simulink model "AAI_VVI"  (R2020a)
settings: Solver=FixedStepAuto  StartTime=0.0  StopTime=10.0  FixedStep=1e-3  RelTol=1e-3  EnableMultiTasking=on
settings Model: NumberOfSteps=10  PacingRate=0.100000  ExtModeTrigDuration=5  Creator=theodor  LastModifiedBy=theodor
settings OptimizationCC: EnhancedBackFolding=on  PassReuseOutputArgsAs=Individual arguments  ZeroExternalMemoryAtStartup=off  ZeroInternalMemoryAtStartup=off  MaxStackSize=64  OptimizeBlockOrder=speed  DifferentSizesBufferReuse=on  OptimizationCustomize=off  EfficientTunableParamExpr=on
settings DebuggingCC: ParameterTunabilityLossMsg=error
settings HardwareCC: ProdBitPerPointer=32  ProdBitPerSizeT=32  ProdBitPerPtrDiffT=32  ProdLargestAtomicInteger=Long  ProdLargestAtomicFloat=Double  ProdWordSize=32  ProdHWDeviceType=ARM Compatible->ARM Cortex
settings SFSimCC: MATLABDynamicMemAlloc=off
settings RTWCC: SystemTargetFile=ert.tlc  HardwareBoard=NXP FRDM-K64F  TemplateMakefile=ert_default_tmf  Toolchain=GNU Tools for ARM Embedded Processors
settings CodeAppCC: ForceParamTrailComments=on  IgnoreCustomStorageClasses=off  OperatorAnnotations=on  SimulinkDataObjDesc=on  SFDataObjDesc=on  InsertBlockDesc=on

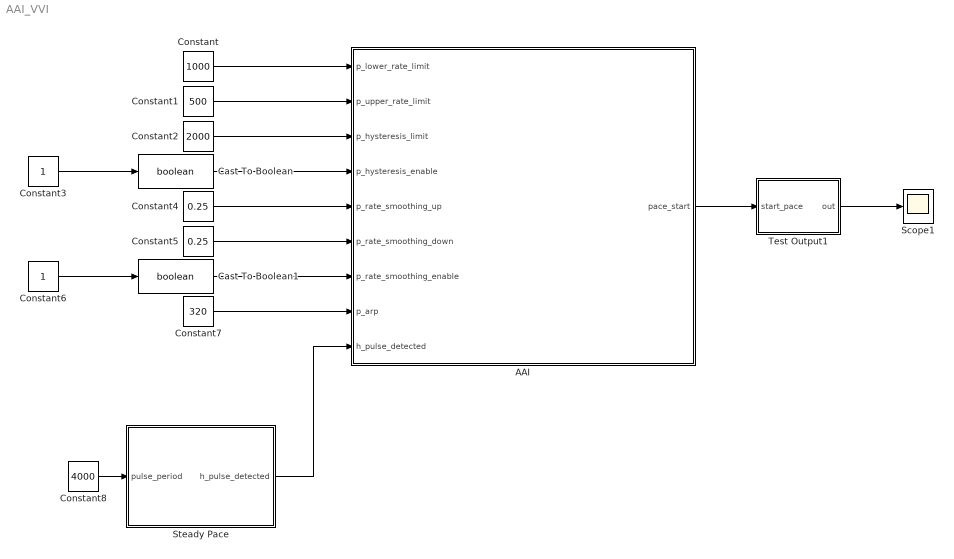
== system AAI_VVI ==
  AAI : Stateflow chart  TreatAsAtomicUnit=on
  Cast To Boolean : DataTypeConversion  OutDataTypeStr=boolean
  Cast To Boolean1 : DataTypeConversion  OutDataTypeStr=boolean
  Constant : Constant  Value=1000
  Constant1 : Constant  Value=500
  Constant2 : Constant  Value=2000
  Constant3 : Constant
  Constant4 : Constant  Value=0.25
  Constant5 : Constant  Value=0.25
  Constant6 : Constant
  Constant7 : Constant  Value=320
  Constant8 : Constant  Value=4000
  Scope1 : Scope
  Steady Pace : Stateflow chart  TreatAsAtomicUnit=on
  Test Output1 : Stateflow chart  TreatAsAtomicUnit=on
  wires:
  Constant/1 -> AAI/1(p_lower_rate_limit)
  Constant1/1 -> AAI/2(p_upper_rate_limit)
  Constant2/1 -> AAI/3(p_hysteresis_limit)
  Constant4/1 -> AAI/5(p_rate_smoothing_up)
  Constant5/1 -> AAI/6(p_rate_smoothing_down)
  Constant7/1 -> AAI/8(p_arp)
  Constant8/1 -> Steady Pace/1(pulse_period)
  Constant3/1 -> Cast To Boolean/1
  Cast To Boolean/1 -> AAI/4(p_hysteresis_enable)
  Constant6/1 -> Cast To Boolean1/1
  Cast To Boolean1/1 -> AAI/7(p_rate_smoothing_enable)
  Test Output1/1(out) -> Scope1/1
  AAI/1(pace_start) -> Test Output1/1(start_pace)
  Steady Pace/1(h_pulse_detected) -> AAI/9(h_pulse_detected)

== stateflow chart AAI_VVI/Steady Pace ==
  state IDLE
    entry:
    h_pulse_detected=false;
  state ON
    entry:
    h_pulse_detected=true;
  (default) -> IDLE
  IDLE -> ON : after(pulse_period-10,msec)
  ON -> IDLE : after(10,msec)
  data: pulse_period input; h_pulse_detected output boolean

== stateflow chart AAI_VVI/AAI ==
  state UPPER_RATE_LIMIT
    entry:
    i_limit = p_upper_rate_limit;
    i_limit = i_limit - p_arp;
    exit: i_last_period = p_arp + elapsed(msec);
  state SENSED
  state LOWER_RATE_LIMIT
    entry:
    i_limit = p_lower_rate_limit;
    i_limit = i_limit - p_arp;
    exit: i_last_period = p_arp + elapsed(msec);
  state INITIAL
    entry:
    i_limit = i_last_period;
  state HYSTERESIS_LIMIT
    entry:
    i_limit = p_hysteresis_limit;
    i_limit = i_limit - p_arp;
    exit: i_last_period = p_arp + elapsed(msec);
  state RATE_SMOOTHING_DOWN
    entry:
    i_limit = i_last_period/(1-p_rate_smoothing_down);
    i_limit = i_limit - p_arp;
    exit: i_last_period = p_arp + elapsed(msec);
  state PACED
    entry:
    pace_start = 1;
    on after(1,msec):
    pace_start = 0;
  state RATE_SMOOTHING_UP
    entry:
    i_limit =  i_last_period/(1+p_rate_smoothing_up);
    i_limit = i_limit - p_arp;
    exit: i_last_period = p_arp + elapsed(msec);
  (junction 89) -> SENSED
  (junction 161) -> (junction 164)
  (junction 151) -> (junction 161) [order 2]
  (junction 164) -> (junction 163)
  (junction 151) -> (junction 158) [order 1] : [p_rate_smoothing_enable]
  (junction 118) -> (junction 151) [order 1] : [p_hysteresis_enable]
  (junction 158) -> (junction 182)
  UPPER_RATE_LIMIT -> (junction 89) [order 1] : [h_pulse_detected]
  (junction 182) -> (junction 184) [order 1] : [i_last_period < p_upper_rate_limit*(1-p_rate_smoothing_down)]
  (junction 184) -> UPPER_RATE_LIMIT
  (junction 88) -> (junction 89)
  (junction 182) -> (junction 168) [order 2]
  (junction 202) -> (junction 184)
  SENSED -> (junction 118) : after(p_arp, msec)
  (junction 118) -> (junction 154) [order 2]
  UPPER_RATE_LIMIT -> (junction 100) [order 2] : after(i_limit, msec)
  (default) -> (junction 193)
  INITIAL -> SENSED [order 2] : [h_pulse_detected]
  (junction 100) -> (junction 101)
  (junction 168) -> (junction 170) [order 1] : [i_last_period < p_hysteresis_limit*(1-p_rate_smoothing_down)]
  (junction 168) -> (junction 187) [order 2]
  (junction 170) -> (junction 173)
  (junction 193) -> INITIAL [order 2] : {i_last_period=p_lower_rate_limit}
  (junction 193) -> INITIAL [order 1] : [p_hysteresis_enable]{i_last_period = p_hysteresis_limit}
  LOWER_RATE_LIMIT -> (junction 88) [order 1] : [h_pulse_detected]
  (junction 87) -> (junction 88)
  (junction 148) -> (junction 144)
  (junction 144) -> LOWER_RATE_LIMIT
  (junction 125) -> (junction 148) [order 2]
  (junction 142) -> (junction 144)
  LOWER_RATE_LIMIT -> (junction 101) [order 2] : after(i_limit, msec)
  (junction 101) -> (junction 102)
  INITIAL -> PACED [order 1] : after(i_limit, msec)
  HYSTERESIS_LIMIT -> (junction 87) [order 1] : [h_pulse_detected]
  (junction 86) -> (junction 87)
  (junction 187) -> (junction 163)
  (junction 163) -> HYSTERESIS_LIMIT
  HYSTERESIS_LIMIT -> (junction 102) [order 2] : after(i_limit, msec)
  (junction 102) -> (junction 103)
  (junction 201) -> (junction 202)
  (junction 199) -> (junction 201)
  RATE_SMOOTHING_DOWN -> (junction 86) [order 1] : [h_pulse_detected]
  (junction 82) -> (junction 86)
  (junction 172) -> (junction 173)
  (junction 173) -> RATE_SMOOTHING_DOWN
  (junction 132) -> (junction 172)
  PACED -> (junction 125) : after(p_arp, msec)
  (junction 154) -> (junction 125)
  RATE_SMOOTHING_DOWN -> (junction 103) [order 2] : after(i_limit, msec)
  (junction 125) -> (junction 197) [order 1] : [p_rate_smoothing_enable]
  (junction 103) -> (junction 104)
  (junction 104) -> PACED
  (junction 197) -> (junction 199) [order 1] : [i_last_period < p_upper_rate_limit*(1-p_rate_smoothing_down)]
  (junction 197) -> (junction 128) [order 2]
  (junction 128) -> (junction 132) [order 1] : [i_last_period < p_lower_rate_limit*(1-p_rate_smoothing_down)]
  (junction 128) -> (junction 135) [order 2]
  RATE_SMOOTHING_UP -> (junction 82) [order 1] : [h_pulse_detected]
  (junction 135) -> RATE_SMOOTHING_UP [order 1] : [i_last_period > p_lower_rate_limit(1+ p_rate_smoothing_up)]
  (junction 135) -> (junction 140) [order 2]
  RATE_SMOOTHING_UP -> (junction 104) [order 2] : after(i_limit, msec)
  (junction 140) -> (junction 142)
  data: p_lower_rate_limit input; p_upper_rate_limit input; p_hysteresis_limit input; p_hysteresis_enable input boolean; p_rate_smoothing_up input; p_rate_smoothing_down input; p_rate_smoothing_enable input boolean; p_arp input; i_limit local; pace_start output; h_pulse_detected input boolean; i_last_period local

== stateflow chart AAI_VVI/Test Output1 ==
  state IDLE
    entry:
    out = 0;
  state ON
    entry:
    out = 1;
  state WAIT_FOR_FALLING_EDGE
    entry:
    out = 0;
  (default) -> IDLE
  IDLE -> ON : [start_pace==1]
  WAIT_FOR_FALLING_EDGE -> IDLE : [start_pace==0]
  ON -> WAIT_FOR_FALLING_EDGE : after(10, msec)
  data: out output; start_pace input
